simulink model "ph_guozai"  (Simulink 6.2)
settings: Solver=ode3  StartTime=0.0  StopTime=2  FixedStep=0.005  RelTol=1e-3
values from neighbouring files (symbols this model uses):
  b22 = 0    [sim_3dof.m]
  b24 = (ph2(ma_cnt,alpha_cnt)-ph1(ma_cnt,alpha_cnt))/(1/57.3)/jy*Q*serf*L    [sim_3dof.m]
  b34 = (Ft-(C2(ma_cnt,alpha_cnt)-C1(ma_cnt,alpha_cnt))/(1/57.3)*Q*serf)/(m*v)    [sim_3dof.m]
  km_h = [0.873387605804 0.909736736815]    [hengce.mat]
  t1_h = [-5.72286727263 -5.49461503945]    [hengce.mat]
  tm_h = [-0.365121120283 -0.348561137688]    [hengce.mat]
  v = sim_3dof_result(count(tf_i),5)    [sim_3dof.m]
  zeta_h = [-0.00997234611163 -0.0099155259514]    [hengce.mat]
settings Model: LastModifiedBy=wangjsh
settings DebuggingCC: SolverPrmCheckMsg=warning

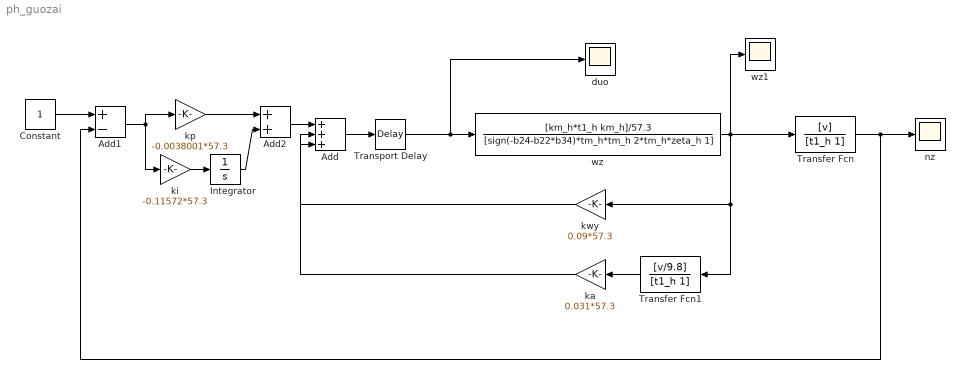
== system ph_guozai ==
  Add : Sum  Inputs=+++  OutScaling=2^-10
  Add1 : Sum  Inputs=+-  OutScaling=2^-10
  Add2 : Sum  OutScaling=2^-10
  Constant : Constant
  Integrator : Integrator
  Transfer Fcn : TransferFcn  Numerator=[v]  Denominator=[t1_h 1]
  Transfer Fcn1 : TransferFcn  Orientation=left  Numerator=[v/9.8]  Denominator=[t1_h 1]
  Transport Delay : TransportDelay  DelayTime=0.05
  duo : Scope
      settings: SaveName=ScopeData2
  ka : Gain  Orientation=left  Gain=0.031*57.3
  ki : Gain  Gain=-0.11572*57.3
  kp : Gain  Gain=-0.0038001*57.3
  kwy : Gain  Orientation=left  Gain=0.09*57.3
  nz : Scope
  wz : TransferFcn  Numerator=[km_h*t1_h km_h]/57.3  Denominator=[sign(-b24-b22*b34)*tm_h*tm_h 2*tm_h*zeta_h 1]
  wz1 : Scope
  wires:
  wz/1 -> wz1/1, Transfer Fcn/1, kwy/1, Transfer Fcn1/1
  Add/1 -> Transport Delay/1
  kwy/1 -> Add/2
  Transfer Fcn/1 -> nz/1, Add1/2
  Constant/1 -> Add1/1
  Add2/1 -> Add/1
  Add1/1 -> kp/1, ki/1
  Integrator/1 -> Add2/2
  kp/1 -> Add2/1
  ki/1 -> Integrator/1
  Transport Delay/1 -> duo/1, wz/1
  ka/1 -> Add/3
  Transfer Fcn1/1 -> ka/1
